simulink model "airport_sim"  (R2021a)
settings: Solver=VariableStepAuto  StartTime=0.0  StopTime=1e7  RelTol=1e-3
undefined symbols (not defined in the file): m, n
settings Model: Creator=hagarusama  LastModifiedBy=hagarusama

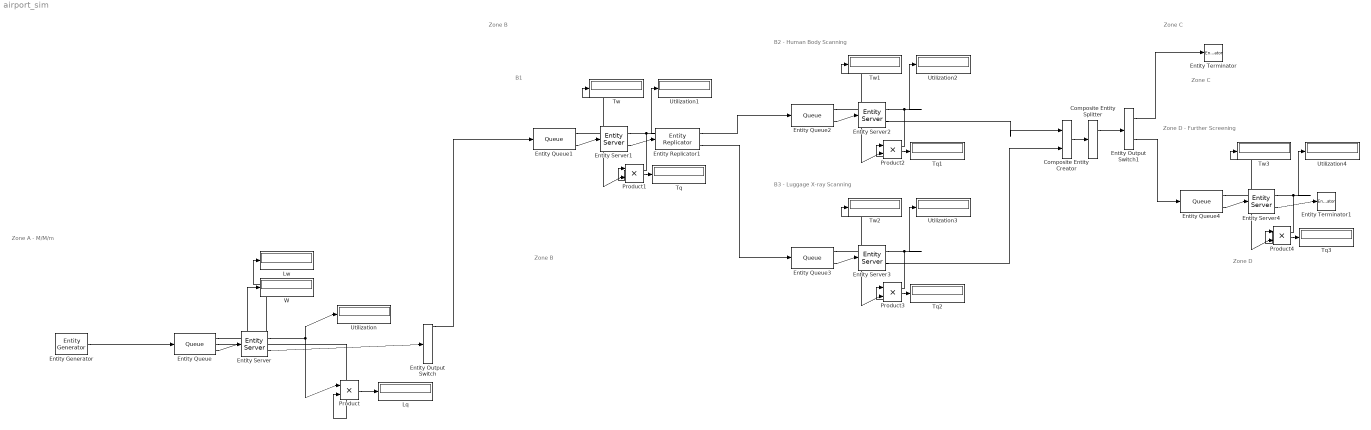
== system airport_sim ==
  note: Zone C
  note: Zone B
  note: Zone B
  note: B1
  note: Zone A - M/M/m
  note: B2 - Human Body Scanning
  note: B3 - Luggage X-ray Scanning
  note: Zone D - Further Screening
  note: Zone C
  note: Zone D
  Composite Entity Creator : CompositeEntityCreator  InputPortMessageModes=m,m  OutputPortMessageModes=m  EntityTypeName=Combined
      settings: InputPortMap=u0,u1
  Composite Entity Splitter : CompositeEntitySplitter  InputPortMessageModes=m  OutputPortMessageModes=m,m
      settings: OutputPortMap=o0,o1
  Entity Output Switch : EntityOutputSwitch  InputPortMessageModes=m  OutputPortMessageModes=m,m,m,m,m  NumberOutputPorts=5  SwitchingCriterion=Equiprobable  Seed=1534953  SwitchAttributeName=Attribute1
      settings: OutputPortMap=o0,o1,o2,o3,o4
  Entity Output Switch1 : EntityOutputSwitch  InputPortMessageModes=m  OutputPortMessageModes=m,m  SwitchingCriterion=Equiprobable  Seed=9631392  SwitchAttributeName=Attribute1
  Entity Generator : EntityGenerator  OutputPortMessageModes=m  TimeSource=MATLAB action  IntergenerationTimeAction=|  EntityType=Structured  EntityTypeName=Entity
      | dt = rand(1,1);
      | persistent rngInit;
      | if isempty(rngInit)
      |     seed = 153503;
      |     rng(seed);
      |     rngInit = true;
      | end
      | 
      | % Pattern: Exponential distribution
      | mu = 3/4;
      | dt = -mu * log(1 - rand());
  Entity Queue{,1..4} (5 alike) : Queue  InputPortMessageModes=m  OutputPortMessageModes=n,n,m  Capacity=inf  AverageWait=on  AverageQueueLength=on
      settings: OutputPortMap=o2,o3,o5
  Entity Replicator1 : EntityReplicator  InputPortMessageModes=m  OutputPortMessageModes=m,m
  Entity Server : EntityServer  InputPortMessageModes=m  OutputPortMessageModes=n,m  ServiceTimeSource=MATLAB action  ServiceTimeAction=|  Utilization=on
      | dt = rand(1,1);
      | persistent rngInit;
      | if isempty(rngInit)
      |     seed = 8084213;
      |     rng(seed);
      |     rngInit = true;
      | end
      | 
      | % Pattern: Exponential distribution
      | mu = 1.2;
      | dt = -mu * log(1 - rand());
      settings: OutputPortMap=o5,o9
  Entity Server1 : EntityServer  InputPortMessageModes=m  OutputPortMessageModes=n,m  Capacity=1  ServiceTimeSource=MATLAB action  ServiceTimeAction=|  Utilization=on
      | dt = rand(1,1);
      | persistent rngInit;
      | if isempty(rngInit)
      |     seed = 2273520;
      |     rng(seed);
      |     rngInit = true;
      | end
      | 
      | % Pattern: Exponential distribution
      | mu = 0.002;
      | dt = -mu * log(1 - rand());
      settings: OutputPortMap=o5,o9
  Entity Server2 : EntityServer  InputPortMessageModes=m  OutputPortMessageModes=n,m  Capacity=1  ServiceTimeSource=MATLAB action  ServiceTimeAction=|  Utilization=on
      | dt = rand(1,1);
      | persistent rngInit;
      | if isempty(rngInit)
      |     seed = 2273520;
      |     rng(seed);
      |     rngInit = true;
      | end
      | 
      | % Pattern: Exponential distribution
      | mu = 0.002;
      | dt = -mu * log(1 - rand());
      settings: OutputPortMap=o5,o9
  Entity Server3 : EntityServer  InputPortMessageModes=m  OutputPortMessageModes=n,m  Capacity=1  ServiceTimeSource=MATLAB action  ServiceTimeAction=|  Utilization=on
      | dt = rand(1,1);
      | persistent rngInit;
      | if isempty(rngInit)
      |     seed = 2273520;
      |     rng(seed);
      |     rngInit = true;
      | end
      | 
      | % Pattern: Exponential distribution
      | mu = 0.002;
      | dt = -mu * log(1 - rand());
      settings: OutputPortMap=o5,o9
  Entity Server4 : EntityServer  InputPortMessageModes=m  OutputPortMessageModes=n,m  Capacity=1  ServiceTimeSource=MATLAB action  ServiceTimeAction=|  Utilization=on
      | dt = rand(1,1);
      | persistent rngInit;
      | if isempty(rngInit)
      |     seed = 2273520;
      |     rng(seed);
      |     rngInit = true;
      | end
      | 
      | % Pattern: Exponential distribution
      | mu = 0.002;
      | dt = -mu * log(1 - rand());
      settings: OutputPortMap=o5,o9
  Entity Terminator : EntityTerminator  InputPortMessageModes=m
  Entity Terminator1 : EntityTerminator  InputPortMessageModes=m
  Lq : Display
  Lw : Display
  Product{,1..4} (5 alike) : Product
  Tq{,1..3} (4 alike) : Display
  Tw{,1..3} (4 alike) : Display
  Utilization{,1..4} (5 alike) : Display
  W : Display
  wires:
  Entity Queue/3 -> Entity Server/1
  Entity Queue/2 -> Product/2, Lw/1
  Entity Queue/1 -> W/1
  Entity Server/1 -> Product/1, Utilization/1
  Product/1 -> Lq/1
  Entity Server/2 -> Entity Output Switch/1
  Entity Generator/1 -> Entity Queue/1
  Entity Server1/2 -> Entity Replicator1/1
  Entity Queue1/3 -> Entity Server1/1
  Entity Server1/1 -> Product1/1, Utilization1/1
  Entity Queue1/1 -> Product1/2, Tw/1
  Product1/1 -> Tq/1
  Product2/1 -> Tq1/1
  Entity Queue2/1 -> Product2/2, Tw1/1
  Entity Server2/1 -> Product2/1, Utilization2/1
  Entity Queue2/3 -> Entity Server2/1
  Entity Queue3/3 -> Entity Server3/1
  Entity Server3/1 -> Product3/1, Utilization3/1
  Entity Queue3/1 -> Product3/2, Tw2/1
  Product3/1 -> Tq2/1
  Entity Replicator1/1 -> Entity Queue2/1
  Entity Output Switch/1 -> Entity Queue1/1
  Entity Replicator1/2 -> Entity Queue3/1
  Product4/1 -> Tq3/1
  Entity Queue4/1 -> Product4/2, Tw3/1
  Entity Server4/1 -> Product4/1, Utilization4/1
  Entity Queue4/3 -> Entity Server4/1
  Entity Server2/2 -> Composite Entity Creator/1
  Entity Server3/2 -> Composite Entity Creator/2
  Composite Entity Creator/1 -> Composite Entity Splitter/1
  Composite Entity Splitter/1 -> Entity Output Switch1/1
  Entity Output Switch1/2 -> Entity Queue4/1
  Entity Output Switch1/1 -> Entity Terminator/1
  Entity Server4/2 -> Entity Terminator1/1
